simulink model "Van_der_Pol_Oscillator"  (R2021b)
settings: Solver=FixedStepAuto  StartTime=0.0  StopTime=531.27  FixedStep=0.01  RelTol=1e-3
undefined symbols (not defined in the file): mu
settings Model: Creator=pagli  LastModifiedBy=pagli

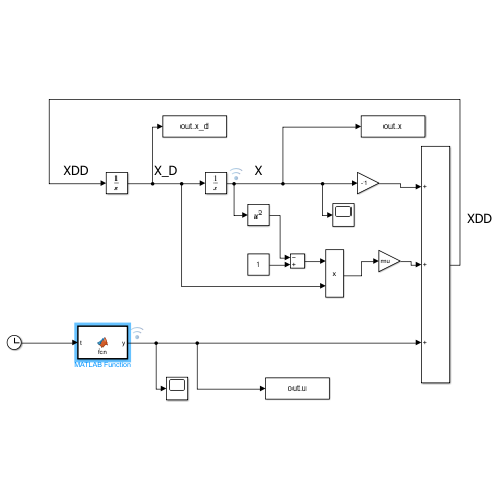
[thumbnail: Simulink's stored preview of the top-level diagram]
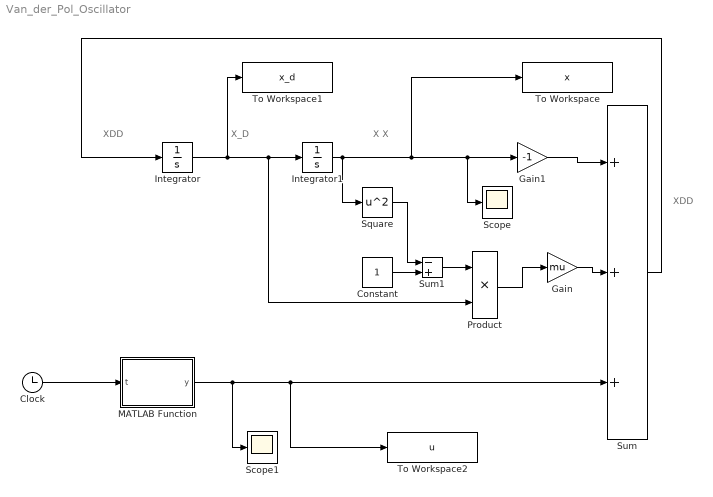
== system Van_der_Pol_Oscillator ==
  note: XDD
  note: X
      | X
  note: XDD
  note: X_D
  Clock : Clock
  Constant : Constant
  Gain : Gain  Gain=mu
  Gain1 : Gain  Gain=-1
  Integrator : Integrator
  Integrator1 : Integrator  InitialCondition=0.1
  MATLAB Function : MATLAB Function  TreatAsAtomicUnit=on
  Product : Product
  Scope : Scope
  Scope1 : Scope
  Square : Math  Operator=square  SaturateOnIntegerOverflow=on
  Sum : Sum  Inputs=+++
  Sum1 : Sum  Inputs=-+
  To Workspace : ToWorkspace  VariableName=x  SampleTime=-1
  To Workspace1 : ToWorkspace  VariableName=x_d  SampleTime=-1
  To Workspace2 : ToWorkspace  VariableName=u  SampleTime=-1
  wires:
  Gain1/1 -> Sum/1
  Sum/1 -> Integrator/1
  Integrator1/1 -> Square/1, To Workspace/1, Scope/1, Gain1/1
  Integrator/1 -> To Workspace1/1, Integrator1/1, Product/2
  Gain/1 -> Sum/2
  Constant/1 -> Sum1/2
  Square/1 -> Sum1/1
  Sum1/1 -> Product/1
  Product/1 -> Gain/1
  MATLAB Function/1(y) -> Scope1/1, To Workspace2/1, Sum/3
  Clock/1 -> MATLAB Function/1(t)

== matlab function Van_der_Pol_Oscillator/MATLAB Function ==
  settings: updateMethod=DISCRETE
  data: t input; y output
function y  = fcn(t) %we don't need (0,0) as initial condition (it is not mandatory). 
                     % Final condition of the previous case can be the initial condition of current case
    y=0;
    train_interval_length = 34.70;
    train_interval_index = floor(t/train_interval_length); %considering t belongs to [0, 451.1 = 13*34.70], then interval_index belongs to [0, 12]
    train_interval_instant = t - (train_interval_index*train_interval_length); %interval_istant belongs to [0, 34.70]
    amplitude = floor(train_interval_instant/6) + 1;
    % Signals for Training Dataset
    switch train_interval_index
        case 0
            y = amplitude*sin(t); %sine wave with variable amplitude
        case 1
            if mod(amplitude, 2) == 0
                i = -0.1;
            else
                i = 0.1; 
            end
            y = i*amplitude*(train_interval_instant); %ramp with variable slope [positive or negative] and start position
        case 2
            y = amplitude*(sin(t)^2);
        case 3
            if amplitude <= 3
                i = 1;
            else
                i = 0; 
            end
            y = i*(train_interval_instant) - (1-i)*(train_interval_instant-train_interval_length-1.2) ;
        case 4
            y = amplitude*square(pi/4*t);
        case 5
            y = amplitude*sawtooth(pi/4*t);
        case 6
            y = amplitude*atan(train_interval_instant);
        case 7
            y = log(train_interval_instant + 1)*sin(t)*cos(t);
        case 8
            y = amplitude*sawtooth(pi/4*t)*sin(t);
        case 9
            y = amplitude*square(pi/4*t)*sin(t);
        case 10
            y = square(pi/4*t)*sqrt(train_interval_instant);
        case 11
            y = 1 - square(pi*t);
        case 12
            y = sqrt(train_interval_instant) - amplitude*square(pi/2*t);
    end

    %Signal for Validation Dataset
    val_interval_length = 20;
    val_interval_index = floor((t - 13*train_interval_length)/val_interval_length); %considering t belongs to [0, 80=4*20], then interval_index belongs to [0, 3]
    val_interval_instant = t - 13*train_interval_length - val_interval_index*val_interval_length; %interval_istant belongs to [0, 1.23]
    switch val_interval_index
        case 0
            linear_interval = linspace(-val_interval_length/2, (val_interval_length+0.01)/2, (val_interval_length+0.01)*100);
            sinc_function = sinc(linear_interval);
            amplitude = 10;
            y = amplitude*sinc_function(floor((val_interval_instant+0.01)*100));
        case 1
            amplitude = 5;
            barthan = barthannwin((val_interval_length+0.01)*100);
            y = amplitude*barthan(floor((val_interval_instant+0.02)*100));
        case 2
            y = cos(val_interval_instant);
        case 3
            amplitude = 2.5;
            y = amplitude*rand;
    end
end
